simulink model "taskt62"  (R2016b)
settings: Solver=VariableStepAuto  StartTime=0.0  StopTime=70.0  RelTol=1e-3
values from neighbouring files (symbols this model uses):
  a = 0.02    [task6_2.m]
  b = 1.3    [task6_2.m]
  d = 10    [task6_2.m]
  gamma1 = 5    [task6_2.m]
  gamma2 = 1    [task6_2.m]
  gamma3 = 1    [task6_2.m]
  r = 35    [task6_2.m]
settings Model: Creator=Kristian  LastModifiedBy=Kristian

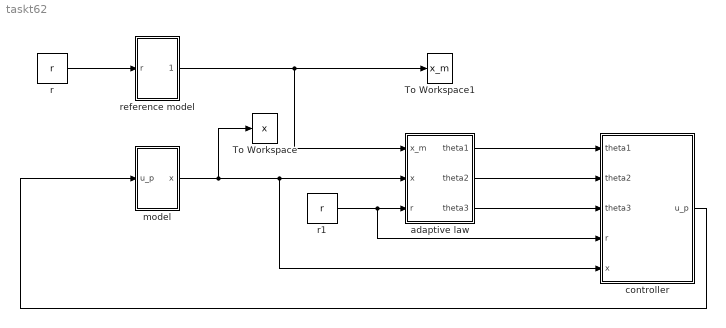
== system taskt62 ==
  To Workspace : ToWorkspace  VariableName=x  SaveFormat=Structure With Time  SampleTime=-1
  To Workspace1 : ToWorkspace  VariableName=x_m  SaveFormat=Structure With Time  SampleTime=-1
  adaptive law : Subsystem
  controller : Subsystem
  model : Subsystem
  r : Constant  Value=r
  r1 : Constant  Value=r
  "reference model " : Subsystem
  wires:
  controller/1(u_p) -> model/1(u_p)
  r/1 -> "reference model "/1(r)
  adaptive law/1(theta1) -> controller/1(theta1)
  adaptive law/2(theta2) -> controller/2(theta2)
  adaptive law/3(theta3) -> controller/3(theta3)
  "reference model "/1(x_m) -> To Workspace1/1, adaptive law/1(x_m)
  model/1(x) -> To Workspace/1, controller/5(x), adaptive law/2(x)
  r1/1 -> controller/4(r), adaptive law/3(r)

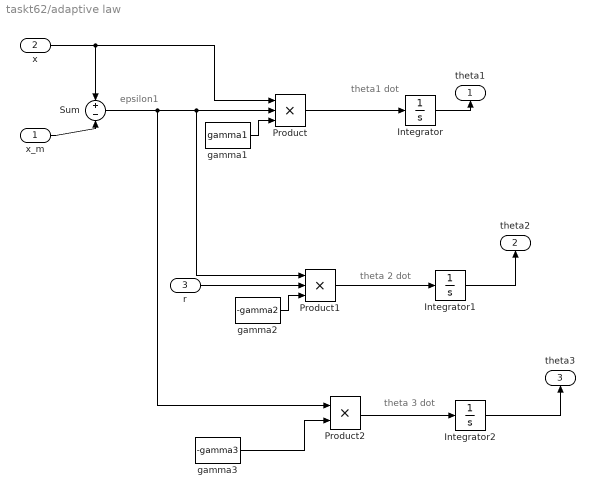
== system taskt62/adaptive law ==
  note: theta 2 dot
  note: theta1 dot
  note: epsilon1
  note: theta 3 dot
  x_m : Inport
  x : Inport  Port=2
  r : Inport  Port=3
  Integrator : Integrator
  Integrator1 : Integrator
  Integrator2 : Integrator
  Product : Product  Inputs=3
  Product1 : Product  Inputs=3
  Product2 : Product
  Sum : Sum  Inputs=+-
  gamma1 : Constant  Value=gamma1
  gamma2 : Constant  Value=-gamma2
  gamma3 : Constant  Value=-gamma3
  theta1 : Outport
  theta2 : Outport  Port=2
  theta3 : Outport  Port=3
  wires:
  x/1 -> Product/1, Sum/1
  x_m/1 -> Sum/2
  Sum/1 -> Product2/1, Product1/1, Product/2
  gamma1/1 -> Product/3
  Product/1 -> Integrator/1
  Integrator/1 -> theta1/1
  gamma2/1 -> Product1/3
  r/1 -> Product1/2
  Product1/1 -> Integrator1/1
  Integrator1/1 -> theta2/1
  gamma3/1 -> Product2/2
  Product2/1 -> Integrator2/1
  Integrator2/1 -> theta3/1

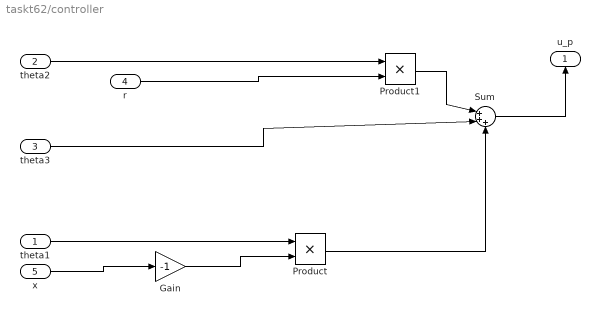
== system taskt62/controller ==
  theta1 : Inport
  theta2 : Inport  Port=2
  theta3 : Inport  Port=3
  r : Inport  Port=4
  x : Inport  Port=5
  Gain : Gain  Gain=-1
  Product : Product
  Product1 : Product
  Sum : Sum  Inputs=|+++
  u_p : Outport
  wires:
  x/1 -> Gain/1
  Gain/1 -> Product/2
  theta2/1 -> Product1/1
  r/1 -> Product1/2
  theta1/1 -> Product/1
  Product1/1 -> Sum/1
  theta3/1 -> Sum/2
  Product/1 -> Sum/3
  Sum/1 -> u_p/1

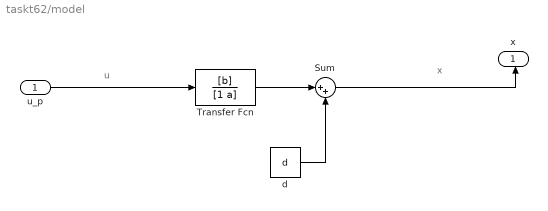
== system taskt62/model ==
  note: x
  note: u
  u_p : Inport
  Sum : Sum  Inputs=|++
  Transfer Fcn : TransferFcn  Numerator=[b]  Denominator=[1 a]
  d : Constant  Value=d
  x : Outport
  wires:
  u_p/1 -> Transfer Fcn/1
  Transfer Fcn/1 -> Sum/1
  d/1 -> Sum/2
  Sum/1 -> x/1

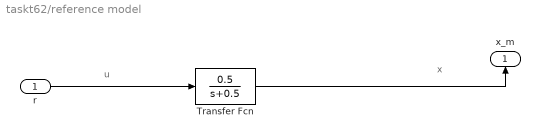
== system taskt62/reference model  ==
  note: x
  note: u
  r : Inport
  Transfer Fcn : TransferFcn  Numerator=[0.5]  Denominator=[1 0.5]
  x_m : Outport
  wires:
  r/1 -> Transfer Fcn/1
  Transfer Fcn/1 -> x_m/1
